simulink model "pitch"  (R2024b)
settings: Solver=VariableStepAuto  StartTime=0.0  StopTime=10.0  RelTol=1e-3
model workspace (MAT data in the model file):
  Ipitch = 2.75e-05
settings Model: Creator=Zohaib  LastModifiedBy=Zohaib

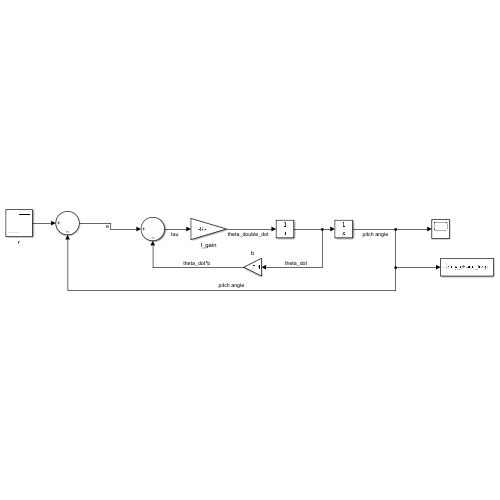
[thumbnail: Simulink's stored preview of the top-level diagram]
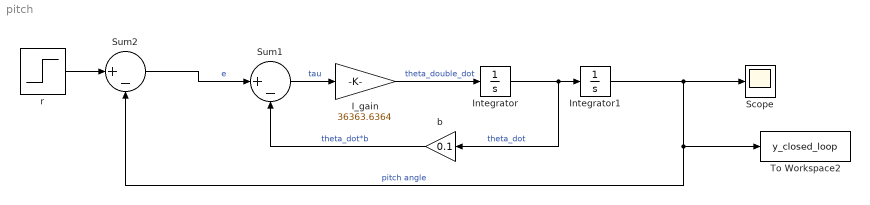
== system pitch ==
  I_gain : Gain  Gain=36363.6364
  Integrator : Integrator
  Integrator1 : Integrator
  Scope : Scope
  Sum1 : Sum  Inputs=|+-
  Sum2 : Sum  Inputs=|+-
  To Workspace2 : ToWorkspace  VariableName=y_closed_loop  SaveFormat=Timeseries  SampleTime=-1
  b : Gain  Gain=0.1
  r : Step  Time=0  SampleTime=0
  wires:
  r/1 -> Sum2/1
  Sum2/1 -> Sum1/1  "e"
  Integrator/1 -> b/1, Integrator1/1  "theta_dot"
  I_gain/1 -> Integrator/1  "theta_double_dot"
  Integrator1/1 -> Scope/1, To Workspace2/1, Sum2/2  "pitch angle"
  Sum1/1 -> I_gain/1  "tau"
  b/1 -> Sum1/2  "theta_dot*b"
